simulink model "paraglider_sim_model_2"  (R2016a)
settings: Solver=VariableStepAuto  StartTime=0.0  StopTime=10.0  RelTol=1e-3
InitFcn:
  | addpath('..');
settings Model: Creator=AkhramovichSA  LastModifiedBy=AkhramovichSA

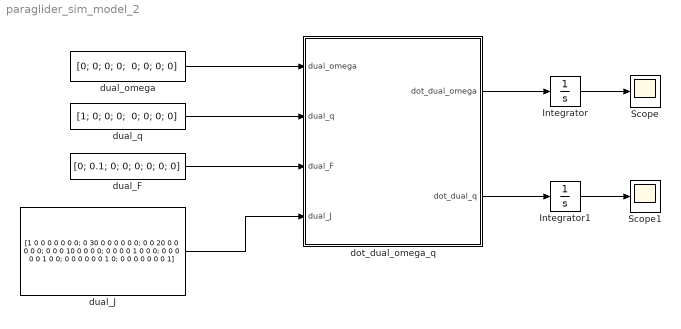
== system paraglider_sim_model_2 ==
  Integrator : Integrator
  Integrator1 : Integrator
  Scope : Scope
  Scope1 : Scope
  dot_dual_omega_q : MATLAB Function  TreatAsAtomicUnit=on
  dual_F : Constant  Value="[0; 0.1; 0; 0;  0; 0; 0; 0]"  VectorParams1D=off
  dual_J : Constant  Value=[1 0 0 0 0 0 0 0; 0 30 0 0 0 0 0 0; 0 0 20 0 0 0 0 0; 0 0 0 10 0 0 0 0; 0 0 0 0 1 0 0 0; 0 0 0 0 0 1 0 0; 0 0 0 0 0 0 1 0; 0 0 0 0 0 0 0 1]  VectorParams1D=off
  dual_omega : Constant  Value="[0; 0; 0; 0;  0; 0; 0; 0]"  VectorParams1D=off
  dual_q : Constant  Value="[1; 0; 0; 0;  0; 0; 0; 0]"  VectorParams1D=off
  wires:
  dual_omega/1 -> dot_dual_omega_q/1(dual_omega)
  dual_q/1 -> dot_dual_omega_q/2(dual_q)
  dual_F/1 -> dot_dual_omega_q/3(dual_F)
  dual_J/1 -> dot_dual_omega_q/4(dual_J)
  dot_dual_omega_q/1(dot_dual_omega) -> Integrator/1
  Integrator/1 -> Scope/1
  dot_dual_omega_q/2(dot_dual_q) -> Integrator1/1
  Integrator1/1 -> Scope1/1

== matlab function paraglider_sim_model_2/dot_dual_omega_q ==
  data: dual_omega input; dot_dual_omega output; dual_q input; dot_dual_q output; dual_F input; dual_J input
function [dot_dual_omega, dot_dual_q] = dot_dual_omega_q(dual_omega, dual_q, dual_F,  dual_J)
% Правые части динамического и кинематического уравнений движения в бикватернионной форме
% Выходные данные надо проинтегрировать звеном: 1/s

% Входные данные:
%
% Бикватернион угловых и линейных скоростей
% dual_omega = [0; omega_x; omega_y; omega_z; 0; v_x; v_y; v_z]
%
% Бикватернион углового и линейного положения
% dual_q     = [q1; q2; q3; q4; q5; q6; q7; q8]
% 
% Бикватернион моментов и сил
% dual_F     = [0; Mx; My; Mz; 0; Fx; Fy; Fz]
%
% Расширенный тензор инерции в бикватернионной форме
% dual_J     = [1  0   0   0  0  0  0  0;
%               0 Jxx Jxy Jxz 0  0  0  0;
%               0 Jyx Jyy Jyz 0  0  0  0;
%               0 Jzx Jzy Jzz 0  0  0  0;
%               0  0   0   0  1  0  0  0;
%               0  0   0   0  0  m  0  0;
%               0  0   0   0  0  0  m  0;
%               0  0   0   0  0  0  0  m]
% 
% Выходные данные:
% 
% Правая часть дифференциального уравнения динамики, изменение бикватерниона угловых и линейных скоростей
% dot_dual_omega = [0; omega_x; omega_y; omega_z; 0; v_x; v_y; v_z]
%
% Правая часть дифференциального уравнения кинематики, изменение бикватерниона углового и линейного положения
% dot_dual_q     = [q1; q2; q3; q4; q5; q6; q7; q8]

dot_dual_omega = dual_J \ (dual_F - dq_cross([dual_omega(1:4); 0; 0; 0; 0], (dual_J*dual_omega))); 

dot_dual_q     = 0.5*dq_multiply(dual_q, dual_omega);
